simulink model "exnb4137986_Q10"  (R2023b)
settings: Solver=FixedStepAuto  StartTime=0  StopTime=100  FixedStep=0.01  RelTol=1e-3
values from neighbouring files (symbols this model uses):
  C = [1 0]    [exnb4137986_Q10.m]
  K2 = place(A3, B, lambda_cl)    [exnb4137986_Q10.m]    (also in exnb4137986_Q9.m)
  Ki = -10    [exnb4137986_Q10.m]
  xeq3 = [5 ... (first row only)    [exnb4137986_Q10.m]    (also in exnb4137986_Q9.m)
libraries: simulink x1
settings Model: Creator=therk  LastModifiedBy=therk

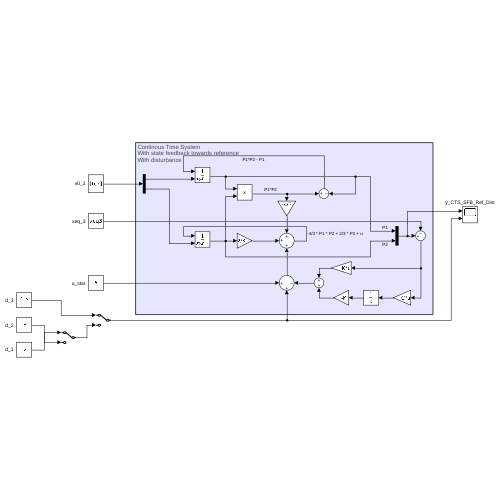
[thumbnail: Simulink's stored preview of the top-level diagram]
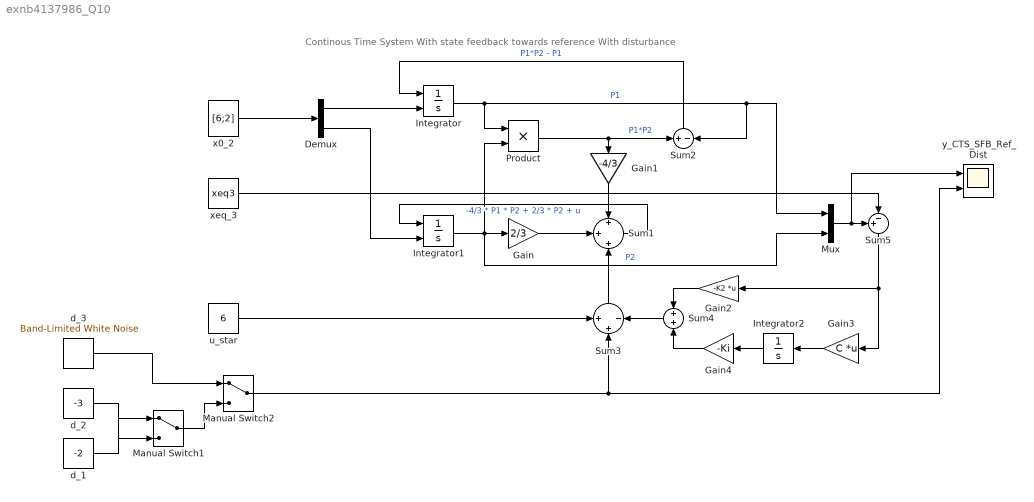
== system exnb4137986_Q10 ==
  note: Continous Time System
      | With state feedback towards reference
      | With disturbance
  Demux : Demux  Outputs=2
  Gain : Gain  Gain=2/3
  Gain1 : Gain  Gain=-4/3
  Gain2 : Gain  Gain=-K2  Multiplication=Matrix(K*u)
  Gain3 : Gain  Gain=C  Multiplication=Matrix(K*u)
  Gain4 : Gain  Gain=-Ki
  Integrator : Integrator  InitialConditionSource=external
  Integrator1 : Integrator  InitialConditionSource=external
  Integrator2 : Integrator
  Manual Switch1 : ManualSwitch
  Manual Switch2 : ManualSwitch
  Mux : Mux  Inputs=2
  Product : Product
  Sum1 : Sum  Inputs=+|+|+
  Sum2 : Sum  Inputs=+|-
  Sum3 : Sum  Inputs=+|+|-
  Sum4 : Sum
  Sum5 : Sum  Inputs=+-|
  d_1 : Constant  Value=-2
  d_2 : Constant  Value=-3
  d_3 : simulink/Sources/Band-Limited White Noise  Cov=[10]  Ts=10  seed=[23341]
  u_star : Constant  Value=6
  x0_2 : Constant  Value=[6;2]
  xeq_3 : Constant  Value=xeq3
  y_CTS_SFB_Ref_Dist : Scope  NumInputPorts=2
  wires:
  Sum4/1 -> Sum3/3
  Integrator1/1 -> Mux/2, Gain/1, Product/2  "P2"
  Gain3/1 -> Integrator2/1
  u_star/1 -> Sum3/1
  Mux/1 -> y_CTS_SFB_Ref_Dist/1, Sum5/1
  Gain4/1 -> Sum4/2
  Sum1/1 -> Integrator1/1  "-4/3 * P1 * P2 + 2/3 * P2 + u"
  Integrator/1 -> Sum2/2, Mux/1, Product/1  "P1"
  Gain/1 -> Sum1/2
  d_1/1 -> Manual Switch1/1
  Gain2/1 -> Sum4/1
  Sum5/1 -> Gain3/1, Gain2/1
  d_2/1 -> Manual Switch1/2
  Integrator2/1 -> Gain4/1
  x0_2/1 -> Demux/1
  Sum3/1 -> Sum1/3
  d_3/1 -> Manual Switch2/1
  Sum2/1 -> Integrator/1  "P1*P2 - P1"
  Manual Switch2/1 -> y_CTS_SFB_Ref_Dist/2, Sum3/2
  Demux/2 -> Integrator1/2
  Manual Switch1/1 -> Manual Switch2/2
  Product/1 -> Sum2/1, Gain1/1  "P1*P2"
  xeq_3/1 -> Sum5/2
  Gain1/1 -> Sum1/1
  Demux/1 -> Integrator/2
